simulink model "pid_nco_pid_mod"  (R2018a)
settings: Solver=VariableStepAuto  StartTime=0.0  StopTime=1  RelTol=1e-3
InitFcn:
  | modelSettings
undefined symbols (not defined in the file): coeff, RadioSampleRate, sps
libraries: simulink x4, RxTxFixedPointLibrary_noscopes_mod x4, commsource2 x1, commdigbbndpm3 x1, dsphdlfiltering x1
settings Model: Creator=czjte  LastModifiedBy=czjte

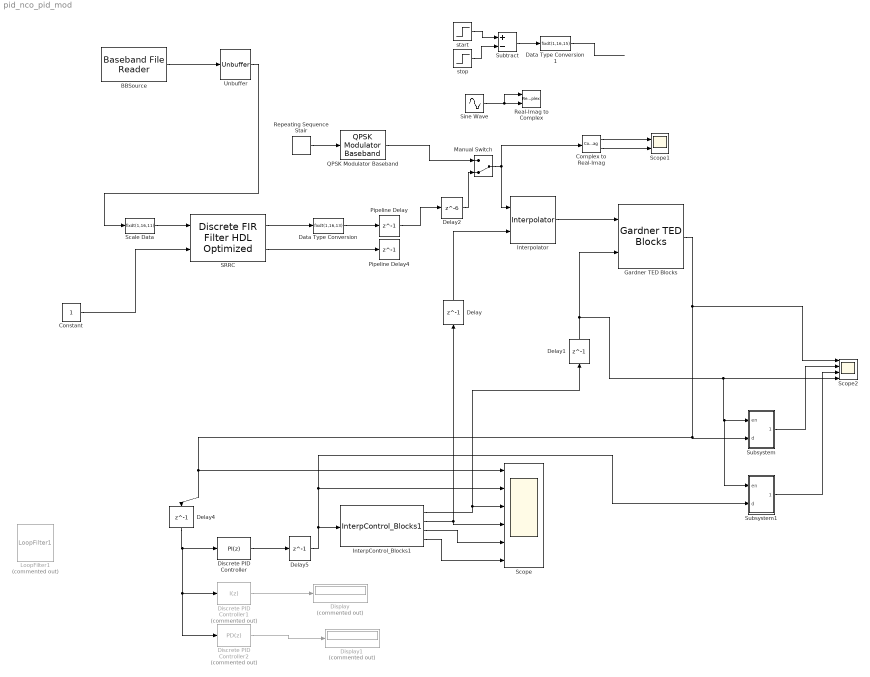
== system pid_nco_pid_mod ==
  BBSource : commsource2/Baseband File Reader  Filename=PlutoCaptureQPSK.bb  InheritSampleTimeFromFile=off  SampleTime=100000/(RadioSampleRate)  SamplesPerFrame=100000  CyclicRepetition=off  FileEndOutputPort=off  SimulateUsing=Interpreted execution
      settings: SourceProductName=Communications System Toolbox  SourceProductBaseCode=CM
  Complex to Real-Imag : ComplexToRealImag
  Constant : Constant  OutDataTypeStr=boolean
  Data Type Conversion : DataTypeConversion  OutDataTypeStr=fixdt(1,16,13)
  Data Type Conversion1 : DataTypeConversion  OutDataTypeStr=fixdt(1,16,15)
  Delay : Delay  DelayLength=1
  Delay1 : Delay  DelayLength=1
  Delay2 : Delay  DelayLength=6
  Delay4 : Delay  DelayLength=1  SampleTime=1/RadioSampleRate
  Delay5 : Delay  DelayLength=1  SampleTime=1/RadioSampleRate
  Discrete PID Controller : simulink/Continuous/PID Controller  Controller=PI  TimeDomain=Discrete-time  SampleTime=1/RadioSampleRate  IntegratorMethod=Forward Euler  FilterMethod=Forward Euler  Form=Parallel  UseFilter=on  ControllerParametersSource=internal  P=-0.004  I=-0.0001  D=-0.00002  N=0.0001  InitialConditionSource=internal  InitialConditionForIntegrator=0  InitialConditionForFilter=0  ExternalReset=none  LimitOutput=off  UpperSaturationLimit=inf  LowerSaturationLimit=-inf  LinearizeAsGain=off  AntiWindupMode=none  Kb=1  TrackingMode=off  Kt=1  PParamMin=[]  PParamMax=[]  IParamMin=[]  IParamMax=[]  DParamMin=[]  DParamMax=[]  NParamMin=[]  NParamMax=[]  KbParamMin=[]  KbParamMax=[]  KtParamMin=[]  KtParamMax=[]  POutMin=[]  POutMax=[]  IOutMin=[]  IOutMax=[]  DOutMin=[]  DOutMax=[]  NOutMin=[]  NOutMax=[]  KbOutMin=[]  KbOutMax=[]  KtOutMin=[]  KtOutMax=[]  IntegratorOutMin=[]  IntegratorOutMax=[]  FilterOutMin=[]  FilterOutMax=[]  FilterOutDataTypeStr=fixdt(1,32,29)  SumOutMin=[]  SumOutMax=[]  SumI1OutMin=[]  SumI1OutMax=[]  SumI2OutMin=[]  SumI2OutMax=[]  SumI3OutMin=[]  SumI3OutMax=[]  SumDOutMin=[]  SumDOutMax=[]  SaturationOutMin=[]  SaturationOutMax=[]  IntegratorContinuousStateAttributes=''  IntegratorStateMustResolveToSignalObject=off  IntegratorRTWStateStorageClass=Auto  FilterContinuousStateAttributes=''  FilterStateMustResolveToSignalObject=off  FilterRTWStateStorageClass=Auto  DifferentiatorICPrevScaledInput=0  DifferentiatorOutMin=[]  DifferentiatorOutMax=[]  FilterDiffOutCoefMin=[]  FilterDiffOutCoefMax=[]  SumDenOutMin=[]  SumDenOutMax=[]  SumNumOutMin=[]  SumNumOutMax=[]  ReciprocalOutMin=[]  ReciprocalOutMax=[]  DivideOutMin=[]  DivideOutMax=[]  TunerSelectOption=Transfer Function Based (PID Tuner App)
  Discrete PID Controller1 : simulink/Continuous/PID Controller  Commented=on  Controller=I  TimeDomain=Discrete-time  SampleTime=1/RadioSampleRate  IntegratorMethod=Forward Euler  FilterMethod=Forward Euler  Form=Parallel  UseFilter=off  ControllerParametersSource=internal  P=-0.003278  I=-0.05  D=0.0  N=6  InitialConditionSource=internal  InitialConditionForIntegrator=0  InitialConditionForFilter=0  ExternalReset=none  LimitOutput=off  UpperSaturationLimit=inf  LowerSaturationLimit=-inf  LinearizeAsGain=off  AntiWindupMode=none  Kb=1  TrackingMode=off  Kt=1  PParamMin=[]  PParamMax=[]  IParamMin=[]  IParamMax=[]  DParamMin=[]  DParamMax=[]  NParamMin=[]  NParamMax=[]  KbParamMin=[]  KbParamMax=[]  KtParamMin=[]  KtParamMax=[]  POutMin=[]  POutMax=[]  IOutMin=[]  IOutMax=[]  DOutMin=[]  DOutMax=[]  NOutMin=[]  NOutMax=[]  KbOutMin=[]  KbOutMax=[]  KtOutMin=[]  KtOutMax=[]  IntegratorOutMin=[]  IntegratorOutMax=[]  FilterOutMin=[]  FilterOutMax=[]  FilterOutDataTypeStr=fixdt(1,32,29)  SumOutMin=[]  SumOutMax=[]  SumOutDataTypeStr=fixdt(1,16,15)  SumI1OutMin=[]  SumI1OutMax=[]  SumI2OutMin=[]  SumI2OutMax=[]  SumI3OutMin=[]  SumI3OutMax=[]  SumDOutMin=[]  SumDOutMax=[]  SaturationOutMin=[]  SaturationOutMax=[]  IntegratorContinuousStateAttributes=''  IntegratorStateMustResolveToSignalObject=off  IntegratorRTWStateStorageClass=Auto  FilterContinuousStateAttributes=''  FilterStateMustResolveToSignalObject=off  FilterRTWStateStorageClass=Auto  DifferentiatorICPrevScaledInput=0  DifferentiatorOutMin=[]  DifferentiatorOutMax=[]  FilterDiffOutCoefMin=[]  FilterDiffOutCoefMax=[]  SumDenOutMin=[]  SumDenOutMax=[]  SumNumOutMin=[]  SumNumOutMax=[]  ReciprocalOutMin=[]  ReciprocalOutMax=[]  DivideOutMin=[]  DivideOutMax=[]  TunerSelectOption=Transfer Function Based (PID Tuner App)
  Discrete PID Controller2 : simulink/Continuous/PID Controller  Commented=on  Controller=PD  TimeDomain=Discrete-time  SampleTime=1/RadioSampleRate  IntegratorMethod=Forward Euler  FilterMethod=Forward Euler  Form=Parallel  UseFilter=off  ControllerParametersSource=internal  P=0  I=0  D=0.0  N=6  InitialConditionSource=internal  InitialConditionForIntegrator=0  InitialConditionForFilter=0  ExternalReset=none  LimitOutput=off  UpperSaturationLimit=inf  LowerSaturationLimit=-inf  LinearizeAsGain=off  AntiWindupMode=none  Kb=1  TrackingMode=off  Kt=1  PParamMin=[]  PParamMax=[]  IParamMin=[]  IParamMax=[]  DParamMin=[]  DParamMax=[]  NParamMin=[]  NParamMax=[]  KbParamMin=[]  KbParamMax=[]  KtParamMin=[]  KtParamMax=[]  POutMin=[]  POutMax=[]  IOutMin=[]  IOutMax=[]  DOutMin=[]  DOutMax=[]  NOutMin=[]  NOutMax=[]  KbOutMin=[]  KbOutMax=[]  KtOutMin=[]  KtOutMax=[]  IntegratorOutMin=[]  IntegratorOutMax=[]  FilterOutMin=[]  FilterOutMax=[]  FilterOutDataTypeStr=fixdt(1,32,29)  SumOutMin=[]  SumOutMax=[]  SumOutDataTypeStr=fixdt(1,16,15)  SumI1OutMin=[]  SumI1OutMax=[]  SumI2OutMin=[]  SumI2OutMax=[]  SumI3OutMin=[]  SumI3OutMax=[]  SumDOutMin=[]  SumDOutMax=[]  SaturationOutMin=[]  SaturationOutMax=[]  IntegratorContinuousStateAttributes=''  IntegratorStateMustResolveToSignalObject=off  IntegratorRTWStateStorageClass=Auto  FilterContinuousStateAttributes=''  FilterStateMustResolveToSignalObject=off  FilterRTWStateStorageClass=Auto  DifferentiatorICPrevScaledInput=0  DifferentiatorOutMin=[]  DifferentiatorOutMax=[]  FilterDiffOutCoefMin=[]  FilterDiffOutCoefMax=[]  SumDenOutMin=[]  SumDenOutMax=[]  SumNumOutMin=[]  SumNumOutMax=[]  ReciprocalOutMin=[]  ReciprocalOutMax=[]  DivideOutMin=[]  DivideOutMax=[]  TunerSelectOption=Transfer Function Based (PID Tuner App)
  Display : Display  Commented=on
  Display1 : Display  Commented=on
  Gardner TED Blocks : RxTxFixedPointLibrary_noscopes_mod/Receiver HDL/Frame Recover/Gardner Timing Recovery/Gardner TED Blocks
  InterpControl_Blocks1 : RxTxFixedPointLibrary_noscopes_mod/Receiver HDL/Frame Recover/Gardner Timing Recovery/InterpControl_Blocks1
  Interpolator : RxTxFixedPointLibrary_noscopes_mod/Receiver HDL/Frame Recover/Gardner Timing Recovery/Interpolator
  LoopFilter1 : RxTxFixedPointLibrary_noscopes_mod/Receiver HDL/Frame Recover/Gardner Timing Recovery/LoopFilter1  Commented=on  zeta=sqrt(2)  BnTs=0.01  Kp=2.7
  Manual Switch : ManualSwitch  CurrentSetting=0
  Pipeline Delay : Delay  DelayLength=1
  Pipeline Delay4 : Delay  DelayLength=1
  QPSK Modulator Baseband : commdigbbndpm3/QPSK Modulator Baseband  InType=Integer  Enc=Gray  Ph=pi/4  outDtype=Fixed-point  outWordLen=16  outUDDataType=sfix(16)  outFracLenMode=User-defined  outFracLen=13  outDataTypeStr=fixdt(1,16,13)  outLastDataTypeStr=fixdt(1,16,13)
  Real-Imag to Complex : RealImagToComplex
  Repeating Sequence Stair : simulink/Sources/Repeating Sequence Stair  OutValues=[0 1 2 3]  tsamp=sps/RadioSampleRate  OutMin=[]  OutMax=[]  OutDataTypeStr=double  OutputDataTypeScalingMode=double  OutDataType=fixdt(0,8)  ConRadixGroup=Best Precision: Vector-wise  OutScaling=2^-12
  SRRC : dsphdlfiltering/Discrete FIR Filter HDL Optimized  Numerator=coeff  Sharing=off  SharingFactor=2  SimulateUsing=Code generation  roundingMode=Floor  overflowMode=on  CoefficientsDataTypeStr=Inherit: Same word length as input  CoefficientsMin=[]  CoefficientsMax=[]  OutputDataTypeStr=fixdt(1,16,11)  OutputMin=[]  OutputMax=[]  ValidInPort=on  ReadyPort=off
      settings: SourceProductName=DSP System Toolbox  SourceProductBaseCode=DS
  Scale Data : DataTypeConversion  OutDataTypeStr=fixdt(1,16,11)  ConvertRealWorld=Stored Integer (SI)  SaturateOnIntegerOverflow=on
  Scope : Scope  NumInputPorts=6
  Scope1 : Scope  NumInputPorts=2
  Scope2 : Scope  NumInputPorts=4
  Sine Wave : Sin  SineType=Sample based  Samples=span  SampleTime=1/RadioSampleRate
  Subsystem : Subsystem
  Subsystem1 : Subsystem
  Subtract : Sum  Inputs=+-
  Unbuffer : Unbuffer
  start : Step  Time=100/RadioSampleRate  After=0.3  SampleTime=1/RadioSampleRate
  stop : Step  Time=1001/RadioSampleRate  After=0  SampleTime=1/RadioSampleRate
  wires:
  InterpControl_Blocks1/1 -> Delay1/1, Scope/3
  InterpControl_Blocks1/2 -> Scope/4, Delay/1
  BBSource/1 -> Unbuffer/1
  SRRC/1 -> Data Type Conversion/1
  Scale Data/1 -> SRRC/1
  Data Type Conversion/1 -> Pipeline Delay/1
  SRRC/2 -> Pipeline Delay4/1
  Pipeline Delay/1 -> Delay2/1
  Interpolator/1 -> Gardner TED Blocks/1
  Delay1/1 -> Scope2/4, Subsystem1/1(en), Subsystem/1(en), Gardner TED Blocks/2
  Delay/1 -> Interpolator/2
  Constant/1 -> SRRC/2
  InterpControl_Blocks1/3 -> Scope/5
  InterpControl_Blocks1/4 -> Scope/6
  Subtract/1 -> Data Type Conversion1/1
  stop/1 -> Subtract/2
  start/1 -> Subtract/1
  Data Type Conversion1/1 -> ?
  Sine Wave/1 -> Real-Imag to Complex/2, Real-Imag to Complex/1
  Repeating Sequence Stair/1 -> QPSK Modulator Baseband/1
  QPSK Modulator Baseband/1 -> Manual Switch/1
  Unbuffer/1 -> Scale Data/1
  Manual Switch/1 -> Complex to Real-Imag/1, Interpolator/1
  Delay2/1 -> Manual Switch/2
  Complex to Real-Imag/1 -> Scope1/1
  Complex to Real-Imag/2 -> Scope1/2
  Gardner TED Blocks/1 -> Delay4/1, Scope/1, Subsystem/2(d), Scope2/1
  Delay4/1 -> Discrete PID Controller2/1, Discrete PID Controller1/1, Discrete PID Controller/1
  Delay5/1 -> Subsystem1/2(d), Scope/2, InterpControl_Blocks1/1
  Discrete PID Controller1/1 -> Display/1
  Discrete PID Controller2/1 -> Display1/1
  Discrete PID Controller/1 -> Delay5/1
  Subsystem/1(cum) -> Scope2/2
  Subsystem1/1(cum) -> Scope2/3

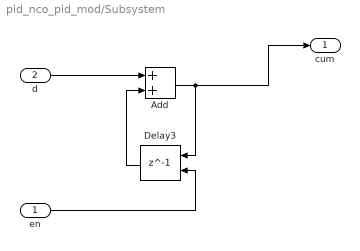
== system pid_nco_pid_mod/Subsystem ==
  en : Inport
  d : Inport  Port=2
  Add : Sum
  Delay3 : Delay  DelayLength=1  ShowEnablePort=on  SampleTime=1/RadioSampleRate
      settings: InputPortMap=u0,e6
  cum : Outport
  wires:
  Add/1 -> cum/1, Delay3/1
  Delay3/1 -> Add/2
  en/1 -> Delay3/2
  d/1 -> Add/1

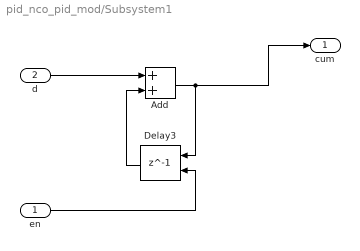
== system pid_nco_pid_mod/Subsystem1 ==
  en : Inport
  d : Inport  Port=2
  Add : Sum
  Delay3 : Delay  DelayLength=1  ShowEnablePort=on  SampleTime=1/RadioSampleRate
      settings: InputPortMap=u0,e6
  cum : Outport
  wires:
  Add/1 -> cum/1, Delay3/1
  Delay3/1 -> Add/2
  en/1 -> Delay3/2
  d/1 -> Add/1
